simulink model "vdPWalker_Belykh_etal_2017"  (R2022a)
settings: Solver=ode4  StartTime=t_inicial_simu  StopTime=t_final_simu  FixedStep=t_step_simu  RelTol=1e-3
values from neighbouring files (symbols this model uses):
  ai = 1    [ImpulseSDOF_1Pedestrian.m]    (also in Impulse_vdpWalkerB2017.m; TeastingvdPWalker_B2017.m; TestingvdPWalker_B2017.m)
  lambdai = 0.23    [ImpulseSDOF_1Pedestrian.m]    (also in Impulse_vdpWalkerB2017.m; TeastingvdPWalker_B2017.m; TestingvdPWalker_B2017.m)
  wi = 0.75    [ImpulseSDOF_1Pedestrian.m]    (also in Impulse_vdpWalkerB2017.m; TeastingvdPWalker_B2017.m = 0.73; TestingvdPWalker_B2017.m)
settings Model: Creator=Javiera  LastModifiedBy=LEGION
settings SolverCC: AlgebraicLoopSolver=TrustRegion
settings DebuggingCC: UnconnectedInputMsg=warning  UnconnectedOutputMsg=warning  UnconnectedLineMsg=warning  SFMachineParentedDataDiag=warning

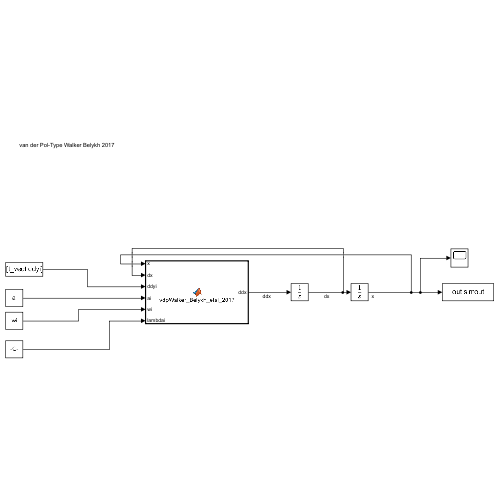
[thumbnail: Simulink's stored preview of the top-level diagram]
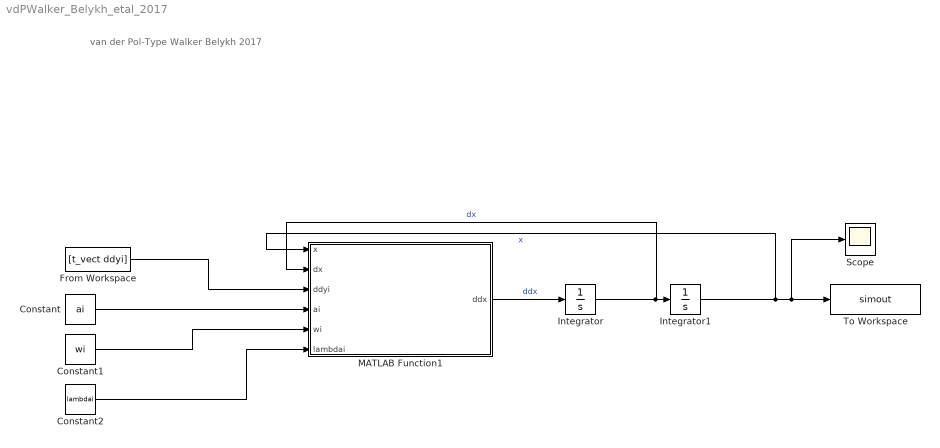
== system vdPWalker_Belykh_etal_2017 ==
  note: van der Pol-Type Walker Belykh 2017
  Constant : Constant  Value=ai
  Constant1 : Constant  Value=wi
  Constant2 : Constant  Value=lambdai
  From Workspace : FromWorkspace  VariableName=[t_vect ddyi]  OutputAfterFinalValue=Setting to zero
  Integrator : Integrator
  Integrator1 : Integrator
  MATLAB Function1 : MATLAB Function  TreatAsAtomicUnit=on
  Scope : Scope
  To Workspace : ToWorkspace  VariableName=simout  SaveFormat=Timeseries  SampleTime=-1
  wires:
  MATLAB Function1/1(ddx) -> Integrator/1  "ddx"
  Integrator/1 -> MATLAB Function1/2(dx), Integrator1/1  "dx"
  Integrator1/1 -> Scope/1, To Workspace/1, MATLAB Function1/1(x)  "x"
  Constant/1 -> MATLAB Function1/4(ai)
  Constant1/1 -> MATLAB Function1/5(wi)
  Constant2/1 -> MATLAB Function1/6(lambdai)
  From Workspace/1 -> MATLAB Function1/3(ddyi)

== matlab function vdPWalker_Belykh_etal_2017/MATLAB Function1 ==
  data: x input; ddx output; dx input; ddyi input; ai input; wi input; lambdai input
function ddx = vdpWalker_Belykh_etal_2017(x,dx,ddyi,ai,wi,lambdai)
% Alexis Contreras R. 

% Foot force models of crowd dynamics on a wobbly bridge
% Igor V. Belykh, Russel Jeter and Vladimir N. Belykh (2017)

% Modelo de peatón de oscilador auto-sostenible donde los pasos se ajustan
% al movimiento del puente. El balance humano se modela como péndulo invertido.
% de la forma de oscilador van der Pol (vdP)

%%%%%%%%%%%%%%%%%%%%%%%%%%%%%%%%%%%%%%%%%%%%%%%%%%%%%%%%%%%%%%%%%%%%%%%%%%%
% Inputs:
% x         -> Desplazamiento del centro de masa (CoM) del peatón
% dx        -> Velocidad del centro de masa del peatón 
% ddyi      -> Aceleración absoluta del puente (o relativa al suelo/punto fijo externo)
% lambdai   -> Parámetro de amortiguamiento
% ai        -> Parámetro de control del mecanismo de auto-excitación del caminar humano
% wi        -> wi = sqrt(g/L), del modelo pendulo invertido (L >> x)

% Outputs:
% ddx       -> Aceleración del peatón
%%%%%%%%%%%%%%%%%%%%%%%%%%%%%%%%%%%%%%%%%%%%%%%%%%%%%%%%%%%%%%%%%%%%%%%%%%%
% fxdx = lambdai*(dx^2-vi^2*x^2+vi^2*ai^2)*dxi-w0^2*xi; (Eq.4)

fxdx = lambdai*(dx^2+x^2*ai^2)*x + wi^2*x;                                  % (Eq.5)
ddx = -ddyi - fxdx;                                                         % (Eq.1)
